simulink model "sampleModel1586"  (R2023a)
settings: Solver=VariableStepAuto  StartTime=0.0  StopTime=10.0  RelTol=1e-3
libraries: hdlsllib x2, simulink x1
settings Model: Creator=user1  LastModifiedBy=user1

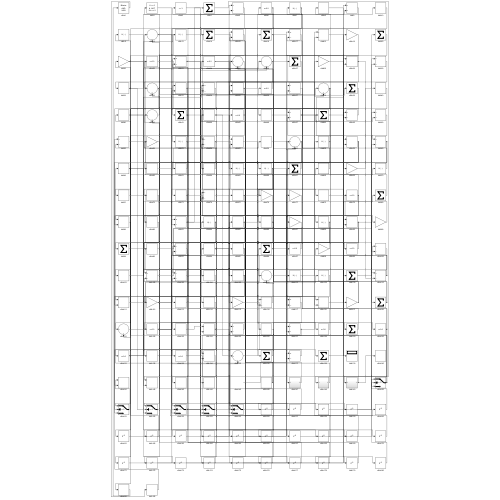
[thumbnail: Simulink's stored preview of the top-level diagram]
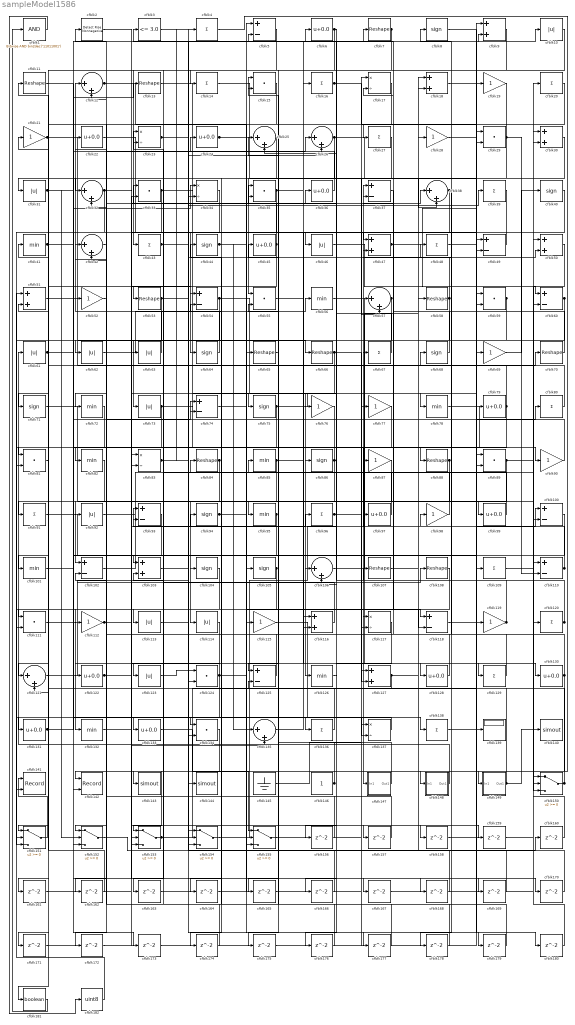
== system sampleModel1586 ==
  cfblk1 : simulink/Logic and Bit Operations/Bitwise Operator  logicop=AND  UseBitMask=on  BitMask=bin2dec('11011001')  BitMaskRealWorld=Stored Integer
      settings: LibrarySourceBlock=|
      | hdlsllib/Logic and Bit
      | Operations/Bitwise
      | Operator
  cfblk{10,31,46,61..63,73,92,113..114,123} (11 alike) : Abs  SaturateOnIntegerOverflow=off
  cfblk{5,37,49,54,60,74,93,100,102,110,118,125} (12 alike) : Sum  Inputs=+-
  cfblk{41,56,72,78,82,85,95,101,126,132} (10 alike) : MinMax
  cfblk{9,18,30,47,50..51,103,116,127} (9 alike) : Sum
  cfblk{8,40,44,64,68,71,75,86,94,104..105} (11 alike) : Signum
  cfblk{12,25..26,32,38,42,57,106,121,135} (10 alike) : Sum  Inputs=|++
  cfblk{7,11,13,53,58,65..66,70,84,88,107..108} (12 alike) : Reshape
  cfblk{4,14,16,20,27,39,43,48,67,80,91,96,109,120,129,136,138} (17 alike) : Sum  Inputs=+
  cfblk{15,29,33,35,55,59,81,89,111,124,134} (11 alike) : DotProduct  OutDataTypeStr=Inherit: Inherit via internal rule
  cfblk{19,21,28,52,69,76..77,87,90,98,112,115,119} (13 alike) : Gain
  cfblk{17,23,34,83,117,137} (6 alike) : Product  Inputs=*/  RndMeth=Zero  SaturateOnIntegerOverflow=on
  cfblk{6,22,24,36,45,79,97,99,122,128,130..131,133} (13 alike) : Bias  Bias=0.0  SaturateOnIntegerOverflow=off
  cfblk139 : Display
  cfblk140 : ToWorkspace  VariableName=simout  SaveFormat=Timeseries  SampleTime=-1
  cfblk141 : Record  FileSettingsInternal="{\"entries\":[{\"content\":{\"excelSettings\":{\"content\":{},\"type\":\"Streamout.ExcelSettings\"}},\"type\":\"Streamout.FileSettingStorage\",\"uuid\":\"\"}],\"packageUris\":[\"http:\\/\\/schema.mathworks.com\\/mf0\\/streamout_blocks\\/R2020a\"],\"version\":\"1.0\"}"  Layout=[1 1]  SignalsInternal="{\"entries\":[{\"content\":{},\"type\":\"RecordBlkView.InputSignals\",\"uuid\":\"\"}],\"packageUris\":[\"http:\\/\\/schema.mathworks.com\\/mf0\\/streamout_blocks\\/R2020a\"],\"version\":\"1.0\"}"  VisualizationBindings="{\"xyplotplugin\":{\"info\":[{\"series\":[{\"bindingParametersList\":[{\"parameter\":\"X-Axis\",\"signalID\":2082,\"signalName\":\"cfblk151\"},{\"parameter\":\"Y-Axis\",\"signalID\":2086,\"signalName\":\"cfblk105\"}],\"seriesID\":54928}],\"subplotID\":1}]}}"  CompatibilityTag=XY  st=-1
  cfblk142 : Record  FileSettingsInternal="{\"entries\":[{\"content\":{\"excelSettings\":{\"content\":{},\"type\":\"Streamout.ExcelSettings\"}},\"type\":\"Streamout.FileSettingStorage\",\"uuid\":\"\"}],\"packageUris\":[\"http:\\/\\/schema.mathworks.com\\/mf0\\/streamout_blocks\\/R2020a\"],\"version\":\"1.0\"}"  Layout=[1 1]  SignalsInternal="{\"entries\":[{\"content\":{},\"type\":\"RecordBlkView.InputSignals\",\"uuid\":\"\"}],\"packageUris\":[\"http:\\/\\/schema.mathworks.com\\/mf0\\/streamout_blocks\\/R2020a\"],\"version\":\"1.0\"}"  VisualizationBindings="{\"xyplotplugin\":{\"info\":[{\"series\":[{\"bindingParametersList\":[{\"parameter\":\"X-Axis\",\"signalID\":2090,\"signalName\":\"cfblk134\"},{\"parameter\":\"Y-Axis\",\"signalID\":2094,\"signalName\":\"cfblk93\"}],\"seriesID\":22479}],\"subplotID\":1}]}}"  CompatibilityTag=XY  st=-1
  cfblk143 : ToWorkspace  VariableName=simout  SaveFormat=Timeseries  SampleTime=-1
  cfblk144 : ToWorkspace  VariableName=simout  SaveFormat=Timeseries  SampleTime=-1
  cfblk145 : Ground
  cfblk146 : Constant  SampleTime=-1
  cfblk147 : Subsystem
      settings: LibrarySourceBlock=|
      | hdlsllib/Ports &
      | Subsystems/Subsystem
  cfblk148 : Subsystem
      settings: LibrarySourceBlock=|
      | hdlsllib/Ports &
      | Subsystems/Subsystem
  cfblk149 : Subsystem
      settings: LibrarySourceBlock=|
      | hdlsllib/Ports &
      | Subsystems/Subsystem
  cfblk{150..155} (6 alike) : Switch  SaturateOnIntegerOverflow=off  InputSameDT=off
  cfblk{156..180} (25 alike) : Delay  SampleTime=1
  cfblk181 : DataTypeConversion  OutDataTypeStr=boolean  SaturateOnIntegerOverflow=off  RndMeth=Floor
  cfblk182 : DataTypeConversion  OutDataTypeStr=uint8  SaturateOnIntegerOverflow=off  RndMeth=Floor
  cfblk2 : hdlsllib/Logic and Bit Operations/Detect Rise Nonnegative  vinit=0  OutDataTypeStr=boolean
  cfblk3 : hdlsllib/Logic and Bit Operations/Compare To Constant  relop=<=  const=3.0  OutDataTypeStr=boolean
  wires:
  cfblk69/1 -> cfblk40/1
  cfblk21/1 -> cfblk70/1, cfblk88/1
  cfblk68/1 -> cfblk37/1
  cfblk110/1 -> cfblk37/2, cfblk48/1
  cfblk51/1 -> cfblk66/1
  cfblk53/1 -> cfblk73/1, cfblk9/2
  cfblk71/1 -> cfblk99/1
  cfblk30/1 -> cfblk55/1
  cfblk121/1 -> cfblk108/1
  cfblk107/1 -> cfblk58/1
  cfblk104/1 -> cfblk132/1
  cfblk4/1 -> cfblk149/1(In1)
  cfblk115/1 -> cfblk138/1
  cfblk59/1 -> cfblk151/2, cfblk175/1, cfblk176/1
  cfblk42/1 -> cfblk2/1
  cfblk99/1 -> cfblk84/1
  cfblk123/1 -> cfblk124/1
  cfblk33/1 -> cfblk90/1, cfblk153/2
  cfblk63/1 -> cfblk12/1
  cfblk83/1 -> cfblk39/1, cfblk4/1
  cfblk78/1 -> cfblk110/1
  cfblk26/1 -> cfblk69/1, cfblk121/2
  cfblk80/1 -> cfblk8/1
  cfblk64/1 -> cfblk52/1
  cfblk56/1 -> cfblk129/1
  cfblk8/1 -> cfblk59/1
  cfblk136/1 -> cfblk21/1
  cfblk84/1 -> cfblk114/1, cfblk163/1
  cfblk90/1 -> cfblk42/1
  cfblk151/1 -> cfblk141/1
  cfblk58/1 -> cfblk7/1, cfblk174/1
  cfblk15/1 -> cfblk62/1
  cfblk148/1(Out1) -> cfblk61/1
  cfblk10/1 -> cfblk95/1
  cfblk131/1 -> cfblk5/2, cfblk74/2
  cfblk79/1 -> cfblk147/1(In1), cfblk125/1, cfblk41/1
  cfblk75/1 -> cfblk78/1, cfblk155/3
  cfblk76/1 -> cfblk126/1
  cfblk73/1 -> cfblk105/1, cfblk81/2
  cfblk82/1 -> cfblk102/1
  cfblk87/1 -> cfblk91/1
  cfblk91/1 -> cfblk139/1
  cfblk150/1 -> cfblk15/1, cfblk35/2
  cfblk66/1 -> cfblk86/1, cfblk118/2, cfblk153/3
  cfblk146/1 -> cfblk45/1, cfblk24/1
  cfblk145/1 -> cfblk17/1
  cfblk62/1 -> cfblk56/1
  cfblk102/1 -> cfblk30/1
  cfblk106/1 -> cfblk28/1
  cfblk9/1 -> cfblk83/2
  cfblk67/1 -> cfblk36/1
  cfblk6/1 -> cfblk43/1, cfblk106/2
  cfblk43/1 -> cfblk103/1, cfblk100/2
  cfblk154/1 -> cfblk97/1
  cfblk130/1 -> cfblk23/1, cfblk153/1, cfblk47/2, cfblk178/1
  cfblk96/1 -> cfblk68/1, cfblk6/1
  cfblk60/1 -> cfblk133/1, cfblk154/3
  cfblk129/1 -> cfblk98/1
  cfblk7/1 -> cfblk53/1, cfblk31/1
  cfblk153/1 -> cfblk29/1, cfblk26/2, cfblk179/1
  cfblk134/1 -> cfblk142/1
  cfblk48/1 -> cfblk79/1
  cfblk29/1 -> cfblk32/1, cfblk27/1, cfblk110/2
  cfblk18/1 -> cfblk119/1
  cfblk13/1 -> cfblk75/1
  cfblk27/1 -> cfblk113/1
  cfblk109/1 -> cfblk20/1
  cfblk55/1 -> cfblk130/1
  cfblk46/1 -> cfblk60/1
  cfblk92/1 -> cfblk49/1
  cfblk120/1 -> cfblk35/1, cfblk17/2
  cfblk125/1 -> cfblk32/2
  cfblk70/1 -> cfblk3/1
  cfblk22/1 -> cfblk116/1
  cfblk137/1 -> cfblk131/1
  cfblk25/1 -> cfblk104/1
  cfblk85/1 -> cfblk67/1, cfblk152/3
  cfblk118/1 -> cfblk80/1
  cfblk149/1(Out1) -> cfblk85/1, cfblk140/1
  cfblk38/1 -> cfblk117/1, cfblk148/1(In1), cfblk121/1
  cfblk35/1 -> cfblk10/1, cfblk143/1
  cfblk112/1 -> cfblk38/1, cfblk135/2
  cfblk34/1 -> cfblk64/1
  cfblk24/1 -> cfblk38/2, cfblk47/1
  cfblk57/1 -> cfblk72/1, cfblk63/1
  cfblk54/1 -> cfblk109/1, cfblk112/1
  cfblk17/1 -> cfblk92/1
  cfblk14/1 -> cfblk57/2
  cfblk77/1 -> cfblk117/2
  cfblk98/1 -> cfblk33/1
  cfblk101/1 -> cfblk34/1
  cfblk39/1 -> cfblk71/1
  cfblk49/1 -> cfblk46/1
  cfblk88/1 -> cfblk116/2, cfblk127/2
  cfblk86/1 -> cfblk136/1, cfblk134/2, cfblk81/1
  cfblk116/1 -> cfblk93/1
  cfblk19/1 -> cfblk101/1
  cfblk2/1 -> cfblk54/1
  cfblk47/1 -> cfblk59/2, cfblk19/1
  cfblk37/1 -> cfblk87/1
  cfblk3/1 -> cfblk144/1
  cfblk72/1 -> cfblk82/1
  cfblk61/1 -> cfblk137/2, cfblk106/1
  cfblk105/1 -> cfblk141/2, cfblk111/1
  cfblk95/1 -> cfblk123/1, cfblk124/2
  cfblk132/1 -> cfblk96/1
  cfblk127/1 -> cfblk18/2, cfblk125/2
  cfblk122/1 -> cfblk128/1, cfblk94/1, cfblk159/1
  cfblk111/1 -> cfblk34/2
  cfblk23/1 -> cfblk89/2, cfblk157/1
  cfblk97/1 -> cfblk44/1
  cfblk89/1 -> cfblk120/1, cfblk134/1, cfblk151/1
  cfblk12/1 -> cfblk115/1, cfblk49/2
  cfblk124/1 -> cfblk122/1, cfblk151/3, cfblk158/1
  cfblk93/1 -> cfblk142/2
  cfblk133/1 -> cfblk155/1
  cfblk94/1 -> cfblk118/1, cfblk177/1
  cfblk119/1 -> cfblk93/2, cfblk25/2
  cfblk31/1 -> cfblk13/1, cfblk11/1, cfblk152/2
  cfblk41/1 -> cfblk26/1, cfblk170/1
  cfblk36/1 -> cfblk12/2
  cfblk32/1 -> cfblk111/2, cfblk167/1
  cfblk103/1 -> cfblk50/2
  cfblk138/1 -> cfblk100/1
  cfblk128/1 -> cfblk107/1
  cfblk52/1 -> cfblk152/1
  cfblk50/1 -> cfblk150/3
  cfblk20/1 -> cfblk155/2
  cfblk16/1 -> cfblk76/1, cfblk29/2
  cfblk147/1(Out1) -> cfblk74/1
  cfblk135/1 -> cfblk16/1
  cfblk5/1 -> cfblk14/1
  cfblk155/1 -> cfblk77/1
  cfblk45/1 -> cfblk22/1, cfblk181/1
  cfblk44/1 -> cfblk65/1, cfblk135/1
  cfblk117/1 -> cfblk156/1
  cfblk156/1 -> cfblk42/2
  cfblk157/1 -> cfblk15/2
  cfblk158/1 -> cfblk150/2
  cfblk159/1 -> cfblk30/2
  cfblk152/1 -> cfblk160/1
  cfblk160/1 -> cfblk50/1
  cfblk81/1 -> cfblk161/1
  cfblk161/1 -> cfblk33/2
  cfblk114/1 -> cfblk162/1
  cfblk162/1 -> cfblk51/2
  cfblk163/1 -> cfblk127/1
  cfblk100/1 -> cfblk164/1
  cfblk164/1 -> cfblk5/1
  cfblk65/1 -> cfblk165/1
  cfblk165/1 -> cfblk137/1
  cfblk126/1 -> cfblk166/1
  cfblk166/1 -> cfblk55/2
  cfblk167/1 -> cfblk60/2
  cfblk113/1 -> cfblk168/1
  cfblk168/1 -> cfblk154/2
  cfblk74/1 -> cfblk169/1
  cfblk169/1 -> cfblk18/1
  cfblk170/1 -> cfblk154/1
  cfblk40/1 -> cfblk171/1
  cfblk171/1 -> cfblk9/1
  cfblk108/1 -> cfblk172/1
  cfblk172/1 -> cfblk83/1
  cfblk11/1 -> cfblk173/1
  cfblk173/1 -> cfblk57/1
  cfblk174/1 -> cfblk102/2
  cfblk175/1 -> cfblk89/1
  cfblk176/1 -> cfblk25/1
  cfblk177/1 -> cfblk23/2
  cfblk178/1 -> cfblk54/2
  cfblk179/1 -> cfblk103/2
  cfblk28/1 -> cfblk180/1
  cfblk180/1 -> cfblk150/1
  cfblk181/1 -> cfblk1/1
  cfblk1/1 -> cfblk182/1
  cfblk182/1 -> cfblk51/1

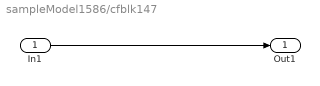
== system sampleModel1586/cfblk147 ==
  In1 : Inport
  Out1 : Outport
  wires:
  In1/1 -> Out1/1

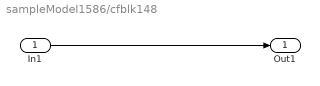
== system sampleModel1586/cfblk148 ==
  In1 : Inport
  Out1 : Outport
  wires:
  In1/1 -> Out1/1

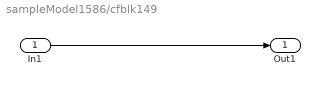
== system sampleModel1586/cfblk149 ==
  In1 : Inport
  Out1 : Outport
  wires:
  In1/1 -> Out1/1
